simulink model "ILCadaptabledoble"  (R2023b)
settings: Solver=VariableStepAuto  StartTime=0.0  StopTime=25  RelTol=1e-3
values from neighbouring files (symbols this model uses):
  BL = 0.00223579    [ILCadaptable.m]    (also in parametros3.m)
  C1 = [1 0 0 0]    [ILCadaptable.m]    (also in parametros3.m = [1 0 0 0 0 0])
  C2 = [0 1 0 0]    [ILCadaptable.m]    (also in parametros3.m = [0 0 1 0 0 0])
  C3 = [0 0 1 0]    [ILCadaptable.m]    (also in parametros3.m = [0 0 0 0 1 0])
  C4 = [0 0 0 1]    [ILCadaptable.m]
  ek1_1 = out.ek1    [ILCadaptable.m]    (also in parametros3.m)
  ek2_1 = out.ek2    [ILCadaptable.m]    (also in parametros3.m)
  JL = 0.00040095    [ILCadaptable.m]    (also in parametros3.m)
  KB = 0.23351629    [ILCadaptable.m]    (also in parametros3.m)
  KD = 5    [ILCadaptable.m]
  KM = 0.23351629    [ILCadaptable.m]    (also in parametros3.m)
  L1 = 2    [ILCadaptable.m]    (also in parametros3.m)
  L2 = 2    [ILCadaptable.m]    (also in parametros3.m)
  LC = 0.0015    [ILCadaptable.m]    (also in parametros3.m)
  RC = 3.4    [ILCadaptable.m]    (also in parametros3.m)
  rt = 10    [ILCadaptable.m]    (also in parametros3.m)
libraries: simulink x2, slpidlib x2
settings Model: Creator=LENOVO  LastModifiedBy=LENOVO

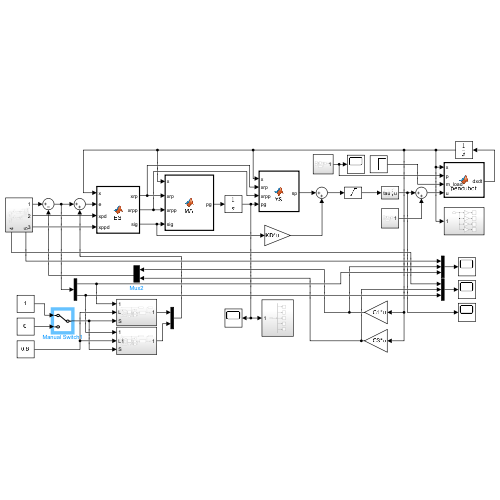
[thumbnail: Simulink's stored preview of the top-level diagram]
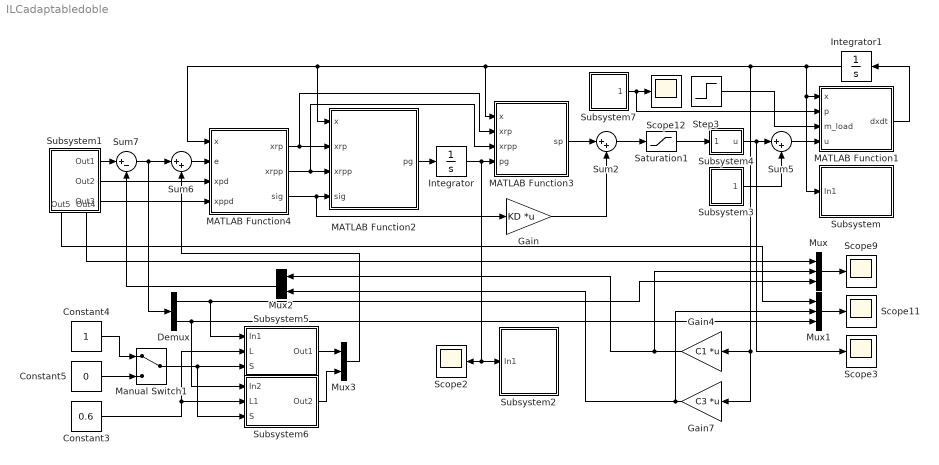
== system ILCadaptabledoble ==
  Constant3 : Constant  Value=0.6
  Constant4 : Constant
  Constant5 : Constant  Value=0
  Demux : Demux  Outputs=2
  Gain : Gain  Gain=KD  Multiplication=Matrix(K*u)
  Gain4 : Gain  Gain=C1  Multiplication=Matrix(K*u)
  Gain7 : Gain  Gain=C3  Multiplication=Matrix(K*u)
  Integrator : Integrator  InitialCondition=[0 0 0 0 0]
  Integrator1 : Integrator  InitialCondition=[-pi/2;0;0;0]
  MATLAB Function1 : MATLAB Function  TreatAsAtomicUnit=on
  MATLAB Function2 : MATLAB Function  TreatAsAtomicUnit=on
  MATLAB Function3 : MATLAB Function  TreatAsAtomicUnit=on
  MATLAB Function4 : MATLAB Function  TreatAsAtomicUnit=on
  Manual Switch1 : ManualSwitch
  Mux : Mux  Inputs=3
  Mux1 : Mux  Inputs=3
  Mux2 : Mux  Inputs=2
  Mux3 : Mux  Inputs=2
  Saturation1 : Saturate  UpperLimit=10  LowerLimit=-10
  Scope{2..3,9,11..12} (5 alike) : Scope
  Step3 : Step  Time=10  After=2  SampleTime=0
  Subsystem : Subsystem
  Subsystem1 : Subsystem
      settings: PortSchema="{\"entries\":[{\"content\":{\"sides\":[{\"content\":{},\"type\":\"ConnectorPlacement.EquallySpacedRectSide\",\"uuid\":\"9b7d0a68-027c-45ca-820c-f278bc6f32a7\"},{\"content\":{\"connectorIds\":[\"Out1\",\"Out2\",\"Out3\"],\"side\":\"RIGHT\"},\"type\":\"ConnectorPlacement.EquallySpacedRectSide\",\"uuid\":\"fa53ec67-4df6-4868-87ee-3d32a2fc1068\"},{\"content\":{\"side\":\"TOP\"},\"type\":\"ConnectorPlacement.EquallySpacedRectSide\",\"uuid\":\"8fcd41cb-9cc9-4cf7-b08f-50ea27c8effa\"},{\"content\":{\"connectorIds\":[\"Out4\",\"Out5\"],\"side\":\"BOTTOM\"},\"type\":\"ConnectorPlacement.EquallySpacedRectSide\",\"uuid\":\"53ef6b28-bc02-4c26-b41f-4cbf5a6224bd\"}]},\"type\":\"ConnectorPlacement.EquallySpacedConnector\",\"uuid\":\"01489902-74b8-4eba-a27b-b5ca226e6d88\"}],\"packageUris\":[\"http://schema.mathworks.com/mf0/Connector/R2020b\"],\"version\":\"1.0\"}"
  Subsystem2 : Subsystem
  Subsystem3 : Subsystem
  Subsystem4 : Subsystem
  Subsystem5 : Subsystem
  Subsystem6 : Subsystem
  Subsystem7 : Subsystem
  Sum2 : Sum  Inputs=|++
  Sum5 : Sum  Inputs=|++
  Sum6 : Sum  Inputs=|++
  Sum7 : Sum  Inputs=|+-
  wires:
  Saturation1/1 -> Subsystem4/1(tau)
  Step3/1 -> MATLAB Function1/3(m_load)
  Gain/1 -> Sum2/2
  MATLAB Function4/3(sig) -> Gain/1, MATLAB Function2/4(sig)
  Sum5/1 -> MATLAB Function1/4(u)
  Sum2/1 -> Saturation1/1
  Subsystem1/5(Out4) -> Mux/1
  Subsystem4/1(u) -> Scope3/1, Sum5/1
  MATLAB Function4/1(xrp) -> MATLAB Function2/2(xrp), MATLAB Function3/2(xrp)
  Mux/1 -> Scope9/1
  Mux1/1 -> Scope11/1
  Subsystem1/2(Out2) -> MATLAB Function4/3(xpd)
  MATLAB Function4/2(xrpp) -> MATLAB Function3/3(xrpp), MATLAB Function2/3(xrpp)
  MATLAB Function1/1(dxdt) -> Integrator1/1
  MATLAB Function3/1(sp) -> Sum2/1
  MATLAB Function2/1(pg) -> Integrator/1
  Subsystem1/4(Out5) -> Mux1/1
  Subsystem1/3(Out3) -> MATLAB Function4/4(xppd)
  Integrator1/1 -> Subsystem/1(In1), MATLAB Function1/1(x), Gain7/1, Gain4/1, MATLAB Function2/1(x), MATLAB Function4/1(x), MATLAB Function3/1(x)
  Integrator/1 -> Subsystem2/1(In1), Scope2/1, MATLAB Function3/4(pg)
  Sum6/1 -> MATLAB Function4/2(e)
  Sum7/1 -> Demux/1, Sum6/1
  Subsystem1/1(Out1) -> Sum7/1
  Constant4/1 -> Manual Switch1/1
  Constant5/1 -> Manual Switch1/2
  Constant3/1 -> Subsystem6/2(L1), Subsystem5/2(L)
  Manual Switch1/1 -> Subsystem6/3(S), Subsystem5/3(S)
  Demux/1 -> Subsystem5/1(In1), Mux/3
  Demux/2 -> Subsystem6/1(In2), Mux1/3
  Mux2/1 -> Sum7/2
  Subsystem5/1(Out1) -> Mux3/1
  Subsystem6/1(Out2) -> Mux3/2
  Mux3/1 -> Sum6/2
  Subsystem7/1(Out1) -> MATLAB Function1/2(p), Scope12/1
  Gain4/1 -> Mux/2, Mux2/1
  Gain7/1 -> Mux1/2, Mux2/2
  Subsystem3/1(Out2) -> Sum5/2

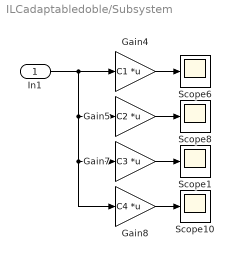
== system ILCadaptabledoble/Subsystem ==
  In1 : Inport
  Gain4 : Gain  Gain=C1  Multiplication=Matrix(K*u)
  Gain5 : Gain  Gain=C2  Multiplication=Matrix(K*u)
  Gain7 : Gain  Gain=C3  Multiplication=Matrix(K*u)
  Gain8 : Gain  Gain=C4  Multiplication=Matrix(K*u)
  Scope{1,6,8,10} (4 alike) : Scope
  wires:
  In1/1 -> Gain8/1, Gain7/1, Gain5/1, Gain4/1
  Gain4/1 -> Scope6/1
  Gain5/1 -> Scope8/1
  Gain7/1 -> Scope1/1
  Gain8/1 -> Scope10/1

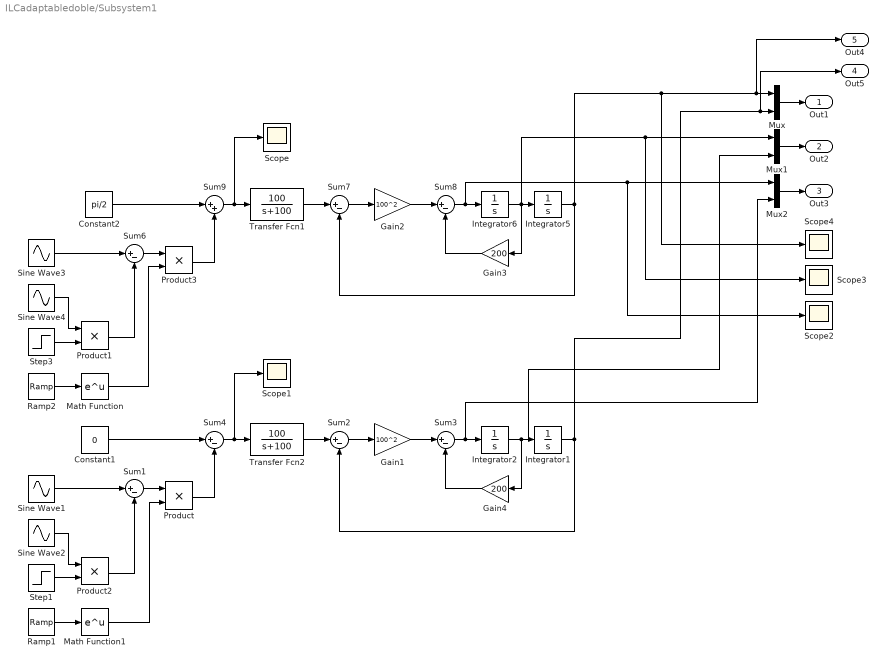
== system ILCadaptabledoble/Subsystem1 ==
  Constant1 : Constant  Value=0
  Constant2 : Constant  Value=pi/2
  Gain1 : Gain  Gain=100^2
  Gain2 : Gain  Gain=100^2
  Gain3 : Gain  Gain=200
  Gain4 : Gain  Gain=200
  Integrator{1..2,5..6} (4 alike) : Integrator
  Math Function : Math
  Math Function1 : Math
  Mux : Mux  Inputs=2
  Mux1 : Mux  Inputs=2
  Mux2 : Mux  Inputs=2
  Product{,1..3} (4 alike) : Product
  Ramp1 : simulink/Sources/Ramp  slope=0  start=10  InitialOutput=0
  Ramp2 : simulink/Sources/Ramp  slope=0  start=10  InitialOutput=0
  Scope{,1..4} (5 alike) : Scope
  Sine Wave1 : Sin  Amplitude=1.4  Frequency=2  SampleTime=0
  Sine Wave2 : Sin  Amplitude=1.4  Frequency=5  SampleTime=0
  Sine Wave3 : Sin  Amplitude=1.4  Frequency=2  SampleTime=0
  Sine Wave4 : Sin  Amplitude=1.4  Frequency=5  SampleTime=0
  Step1 : Step  Time=0  After=0  SampleTime=0
  Step3 : Step  Time=0  After=0  SampleTime=0
  Sum{1..4,6..8} (7 alike) : Sum  Inputs=|+-
  Sum9 : Sum  Inputs=|++
  Transfer Fcn1 : TransferFcn  Numerator=[100]  Denominator=[1 100]
  Transfer Fcn2 : TransferFcn  Numerator=[100]  Denominator=[1 100]
  Out1 : Outport
  Out2 : Outport  Port=2
  Out3 : Outport  Port=3
  Out5 : Outport  Port=4
  Out4 : Outport  Port=5
  wires:
  Mux/1 -> Out1/1
  Mux1/1 -> Out2/1
  Mux2/1 -> Out3/1
  Integrator5/1 -> Scope4/1, Out4/1, Mux/1, Sum7/2
  Sine Wave3/1 -> Sum6/1
  Sum7/1 -> Gain2/1
  Sum8/1 -> Scope2/1, Mux2/1, Integrator6/1
  Sine Wave4/1 -> Product1/1
  Gain2/1 -> Sum8/1
  Transfer Fcn1/1 -> Sum7/1
  Gain3/1 -> Sum8/2
  Product1/1 -> Sum6/2
  Step3/1 -> Product1/2
  Constant2/1 -> Sum9/1
  Integrator6/1 -> Scope3/1, Mux1/1, Gain3/1, Integrator5/1
  Sum9/1 -> Scope/1, Transfer Fcn1/1
  Sum4/1 -> Scope1/1, Transfer Fcn2/1
  Sum3/1 -> Mux2/2, Integrator2/1
  Gain1/1 -> Sum3/1
  Transfer Fcn2/1 -> Sum2/1
  Sum2/1 -> Gain1/1
  Step1/1 -> Product2/2
  Constant1/1 -> Sum4/1
  Integrator1/1 -> Out5/1, Mux/2, Sum2/2
  Sine Wave1/1 -> Sum1/1
  Gain4/1 -> Sum3/2
  Integrator2/1 -> Mux1/2, Gain4/1, Integrator1/1
  Product2/1 -> Sum1/2
  Sine Wave2/1 -> Product2/1
  Math Function/1 -> Product3/2
  Math Function1/1 -> Product/2
  Ramp2/1 -> Math Function/1
  Ramp1/1 -> Math Function1/1
  Sum6/1 -> Product3/1
  Product3/1 -> Sum9/2
  Sum1/1 -> Product/1
  Product/1 -> Sum4/2

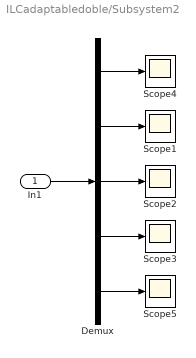
== system ILCadaptabledoble/Subsystem2 ==
  In1 : Inport
  Demux : Demux  Outputs=5
  Scope{1..5} (5 alike) : Scope
  wires:
  In1/1 -> Demux/1
  Demux/3 -> Scope2/1
  Demux/2 -> Scope1/1
  Demux/1 -> Scope4/1
  Demux/4 -> Scope3/1
  Demux/5 -> Scope5/1

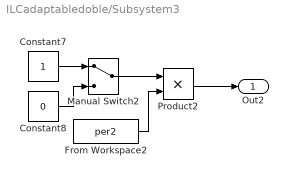
== system ILCadaptabledoble/Subsystem3 ==
  Constant7 : Constant
  Constant8 : Constant  Value=0
  From Workspace2 : FromWorkspace  VariableName=per2
  Manual Switch2 : ManualSwitch
  Product2 : Product
  Out2 : Outport
  wires:
  Product2/1 -> Out2/1
  From Workspace2/1 -> Product2/2
  Constant7/1 -> Manual Switch2/1
  Constant8/1 -> Manual Switch2/2
  Manual Switch2/1 -> Product2/1

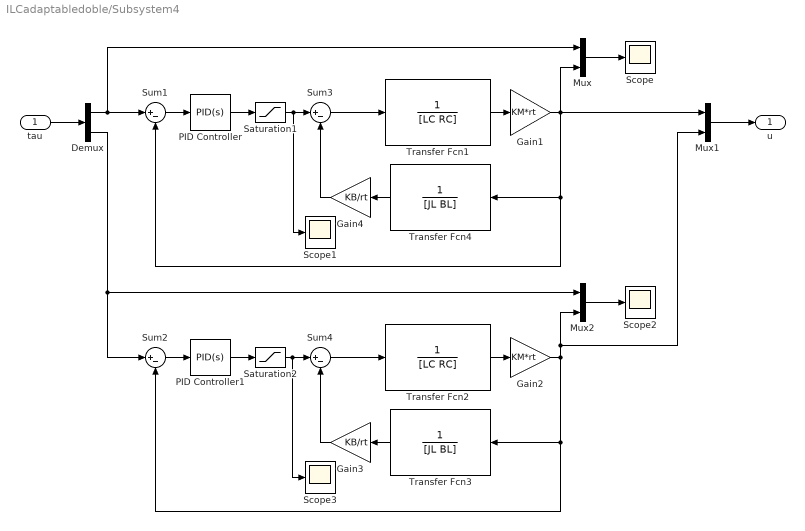
== system ILCadaptabledoble/Subsystem4 ==
  tau : Inport
  Demux : Demux  Outputs=2
  Gain1 : Gain  Gain=KM*rt
  Gain2 : Gain  Gain=KM*rt
  Gain3 : Gain  Gain=KB/rt
  Gain4 : Gain  Gain=KB/rt
  Mux : Mux  Inputs=2
  Mux1 : Mux  Inputs=2
  Mux2 : Mux  Inputs=2
  PID Controller : slpidlib/PID Controller  Controller=PID  Form=Parallel  TimeDomain=Continuous-time  UseExternalTs=off  SampleTime=-1  IntegratorMethod=Forward Euler  FilterMethod=Forward Euler  ControllerParametersSource=internal  P=100  I=50  UseKiTs=off  D=20  N=100  UseFilter=on  TunerSelectOption=Transfer Function Based (PID Tuner App)  InitialConditionSource=internal  InitialConditionForIntegrator=0  InitialConditionForFilter=0  DifferentiatorICPrevScaledInput=0  ExternalReset=none  TrackingMode=off  Kt=1  LimitOutput=off  SatLimitsSource=internal  UpperSaturationLimit=inf  LowerSaturationLimit=-inf  LinearizeAsGain=on  AntiWindupMode=none  Kb=1  LimitIntegrator=off  UpperIntegratorSaturationLimit=inf  LowerIntegratorSaturationLimit=-inf  POutMin=[]  POutMax=[]  IOutMin=[]  IOutMax=[]  DOutMin=[]  DOutMax=[]  NOutMin=[]  NOutMax=[]  SumOutMin=[]  SumOutMax=[]  SaturationOutMin=[]  SaturationOutMax=[]  PParamMin=[]  PParamMax=[]  IParamMin=[]  IParamMax=[]  DParamMin=[]  DParamMax=[]  NParamMin=[]  NParamMax=[]  KbParamMin=[]  KbParamMax=[]  KtParamMin=[]  KtParamMax=[]  KbOutMin=[]  KbOutMax=[]  KtOutMin=[]  KtOutMax=[]  IntegratorOutMin=[]  IntegratorOutMax=[]  FilterOutMin=[]  FilterOutMax=[]  SumI1OutMin=[]  SumI1OutMax=[]  SumI2OutMin=[]  SumI2OutMax=[]  SumI3OutMin=[]  SumI3OutMax=[]  SumI4OutMin=[]  SumI4OutMax=[]  SumDOutMin=[]  SumDOutMax=[]  DifferentiatorOutMin=[]  DifferentiatorOutMax=[]  FilterDiffOutCoefMin=[]  FilterDiffOutCoefMax=[]  ReciprocalOutMin=[]  ReciprocalOutMax=[]  SumDenOutMin=[]  SumDenOutMax=[]  SumNumOutMin=[]  SumNumOutMax=[]  DivideOutMin=[]  DivideOutMax=[]  UdiffTsProdOutMin=[]  UdiffTsProdOutMax=[]  NTsProdOutMin=[]  NTsProdOutMax=[]  UintegralTsProdOutMin=[]  UintegralTsProdOutMax=[]  UngainTsProdOutMin=[]  UngainTsProdOutMax=[]  ClampingZeroOutDataTypeStr=Inherit: Inherit via back propagation  ClampingZeroOutMin=[]  ClampingZeroOutMax=[]  FilterDenConstantOutDataTypeStr=Inherit: Inherit via back propagation  FilterDenConstantOutMin=[]  FilterDenConstantOutMax=[]  PCopyOutDataTypeStr=Inherit: Inherit via back propagation  PCopyOutMin=[]  PCopyOutMax=[]  NCopyOutDataTypeStr=Inherit: Inherit via back propagation  NCopyOutMin=[]  NCopyOutMax=[]  IntegratorContinuousStateAttributes=''  IntegratorStateMustResolveToSignalObject=off  IntegratorRTWStateStorageClass=Auto  FilterContinuousStateAttributes=''  FilterStateMustResolveToSignalObject=off  FilterRTWStateStorageClass=Auto  ParallelPVariant=InternalParameters  IdealPVariant=Disabled  IVariant=InternalParameters  DVariant=InternalParameters  IntegratorVariant=Continuous  SatVariant=Disabled  AWVariant=Passthrough  PCopyVariant=Disabled  TRVariant=Disabled  FdbkBlocksVariant=Forward  IdealPFdbkVariant=Disabled  SatFdbkVariant=Disabled  DerivativeFilterVariant=ContFilter  NVariant=InternalParameters  NCopyVariant=Disabled  FilterICVariant=InternalICsFilter  IntegratorICVariant=InternalICs  ExternalResetVariant=Disabled  TRSumVariant=Passthrough  SumFdbkVariant=Disabled  SumVariant=Sum_PID  TsampFilterVariant=InternalTs  TsampNgainVariant=Passthrough  TsampIntegralVariant=Disabled_SignalSpec  ExternalSaturationOutDataTypeStr=Inherit: Same as second input
  PID Controller1 : slpidlib/PID Controller  Controller=PID  Form=Parallel  TimeDomain=Continuous-time  UseExternalTs=off  SampleTime=-1  IntegratorMethod=Forward Euler  FilterMethod=Forward Euler  ControllerParametersSource=internal  P=100  I=50  UseKiTs=off  D=20  N=100  UseFilter=on  TunerSelectOption=Transfer Function Based (PID Tuner App)  InitialConditionSource=internal  InitialConditionForIntegrator=0  InitialConditionForFilter=0  DifferentiatorICPrevScaledInput=0  ExternalReset=none  TrackingMode=off  Kt=1  LimitOutput=off  SatLimitsSource=internal  UpperSaturationLimit=inf  LowerSaturationLimit=-inf  LinearizeAsGain=on  AntiWindupMode=none  Kb=1  LimitIntegrator=off  UpperIntegratorSaturationLimit=inf  LowerIntegratorSaturationLimit=-inf  POutMin=[]  POutMax=[]  IOutMin=[]  IOutMax=[]  DOutMin=[]  DOutMax=[]  NOutMin=[]  NOutMax=[]  SumOutMin=[]  SumOutMax=[]  SaturationOutMin=[]  SaturationOutMax=[]  PParamMin=[]  PParamMax=[]  IParamMin=[]  IParamMax=[]  DParamMin=[]  DParamMax=[]  NParamMin=[]  NParamMax=[]  KbParamMin=[]  KbParamMax=[]  KtParamMin=[]  KtParamMax=[]  KbOutMin=[]  KbOutMax=[]  KtOutMin=[]  KtOutMax=[]  IntegratorOutMin=[]  IntegratorOutMax=[]  FilterOutMin=[]  FilterOutMax=[]  SumI1OutMin=[]  SumI1OutMax=[]  SumI2OutMin=[]  SumI2OutMax=[]  SumI3OutMin=[]  SumI3OutMax=[]  SumI4OutMin=[]  SumI4OutMax=[]  SumDOutMin=[]  SumDOutMax=[]  DifferentiatorOutMin=[]  DifferentiatorOutMax=[]  FilterDiffOutCoefMin=[]  FilterDiffOutCoefMax=[]  ReciprocalOutMin=[]  ReciprocalOutMax=[]  SumDenOutMin=[]  SumDenOutMax=[]  SumNumOutMin=[]  SumNumOutMax=[]  DivideOutMin=[]  DivideOutMax=[]  UdiffTsProdOutMin=[]  UdiffTsProdOutMax=[]  NTsProdOutMin=[]  NTsProdOutMax=[]  UintegralTsProdOutMin=[]  UintegralTsProdOutMax=[]  UngainTsProdOutMin=[]  UngainTsProdOutMax=[]  ClampingZeroOutDataTypeStr=Inherit: Inherit via back propagation  ClampingZeroOutMin=[]  ClampingZeroOutMax=[]  FilterDenConstantOutDataTypeStr=Inherit: Inherit via back propagation  FilterDenConstantOutMin=[]  FilterDenConstantOutMax=[]  PCopyOutDataTypeStr=Inherit: Inherit via back propagation  PCopyOutMin=[]  PCopyOutMax=[]  NCopyOutDataTypeStr=Inherit: Inherit via back propagation  NCopyOutMin=[]  NCopyOutMax=[]  IntegratorContinuousStateAttributes=''  IntegratorStateMustResolveToSignalObject=off  IntegratorRTWStateStorageClass=Auto  FilterContinuousStateAttributes=''  FilterStateMustResolveToSignalObject=off  FilterRTWStateStorageClass=Auto  ParallelPVariant=InternalParameters  IdealPVariant=Disabled  IVariant=InternalParameters  DVariant=InternalParameters  IntegratorVariant=Continuous  SatVariant=Disabled  AWVariant=Passthrough  PCopyVariant=Disabled  TRVariant=Disabled  FdbkBlocksVariant=Forward  IdealPFdbkVariant=Disabled  SatFdbkVariant=Disabled  DerivativeFilterVariant=ContFilter  NVariant=InternalParameters  NCopyVariant=Disabled  FilterICVariant=InternalICsFilter  IntegratorICVariant=InternalICs  ExternalResetVariant=Disabled  TRSumVariant=Passthrough  SumFdbkVariant=Disabled  SumVariant=Sum_PID  TsampFilterVariant=InternalTs  TsampNgainVariant=Passthrough  TsampIntegralVariant=Disabled_SignalSpec  ExternalSaturationOutDataTypeStr=Inherit: Same as second input
  Saturation1 : Saturate  UpperLimit=250  LowerLimit=-250
  Saturation2 : Saturate  UpperLimit=250  LowerLimit=-250
  Scope{,1..3} (4 alike) : Scope
  Sum{1..4} (4 alike) : Sum  Inputs=|+-
  Transfer Fcn1 : TransferFcn  Denominator=[LC RC]
  Transfer Fcn2 : TransferFcn  Denominator=[LC RC]
  Transfer Fcn3 : TransferFcn  Denominator=[JL BL]
  Transfer Fcn4 : TransferFcn  Denominator=[JL BL]
  u : Outport
  wires:
  tau/1 -> Demux/1
  Demux/1 -> Sum1/1, Mux/1
  Mux/1 -> Scope/1
  Sum1/1 -> PID Controller/1
  Transfer Fcn1/1 -> Gain1/1
  Gain1/1 -> Sum1/2, Transfer Fcn4/1, Mux1/1, Mux/2
  Gain4/1 -> Sum3/2
  Sum3/1 -> Transfer Fcn1/1
  Transfer Fcn4/1 -> Gain4/1
  Mux1/1 -> u/1
  PID Controller/1 -> Saturation1/1
  PID Controller1/1 -> Saturation2/1
  Sum2/1 -> PID Controller1/1
  Demux/2 -> Sum2/1, Mux2/1
  Transfer Fcn2/1 -> Gain2/1
  Transfer Fcn3/1 -> Gain3/1
  Gain3/1 -> Sum4/2
  Gain2/1 -> Mux2/2, Mux1/2, Sum2/2, Transfer Fcn3/1
  Mux2/1 -> Scope2/1
  Sum4/1 -> Transfer Fcn2/1
  Saturation1/1 -> Scope1/1, Sum3/1
  Saturation2/1 -> Scope3/1, Sum4/1

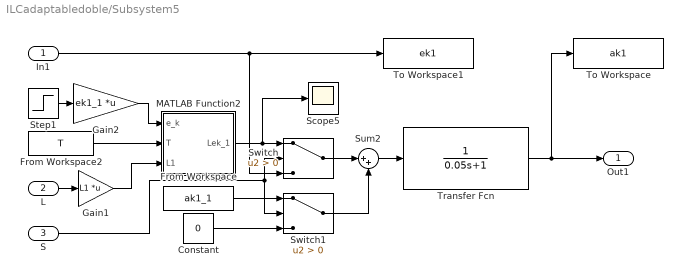
== system ILCadaptabledoble/Subsystem5 ==
  In1 : Inport
  L : Inport  Port=2
  S : Inport  Port=3
  Constant : Constant  Value=0
  From Workspace : FromWorkspace  VariableName=ak1_1
  From Workspace2 : FromWorkspace  VariableName=T
  Gain1 : Gain  Gain=L1  Multiplication=Matrix(K*u)
  Gain2 : Gain  Gain=ek1_1  Multiplication=Matrix(K*u)
  MATLAB Function2 : MATLAB Function  TreatAsAtomicUnit=on
  Scope5 : Scope
  Step1 : Step  Time=0  SampleTime=0
  Sum2 : Sum  Inputs=|++
  Switch : Switch  Criteria=u2 > Threshold  SaturateOnIntegerOverflow=off  InputSameDT=off
  Switch1 : Switch  Criteria=u2 > Threshold  SaturateOnIntegerOverflow=off  InputSameDT=off
  To Workspace : ToWorkspace  VariableName=ak1  SampleTime=-1
  To Workspace1 : ToWorkspace  VariableName=ek1  SampleTime=-1
  Transfer Fcn : TransferFcn  Denominator=[0.05 1]
  Out1 : Outport
  wires:
  From Workspace2/1 -> MATLAB Function2/2(T)
  In1/1 -> Switch/3, To Workspace1/1
  Gain2/1 -> MATLAB Function2/1(e_k)
  Step1/1 -> Gain2/1
  Constant/1 -> Switch1/3
  MATLAB Function2/1(Lek_1) -> Scope5/1, Switch/1
  Sum2/1 -> Transfer Fcn/1
  Switch1/1 -> Sum2/2
  From Workspace/1 -> Switch1/1
  Switch/1 -> Sum2/1
  Transfer Fcn/1 -> To Workspace/1, Out1/1
  L/1 -> Gain1/1
  S/1 -> Switch1/2, Switch/2
  Gain1/1 -> MATLAB Function2/3(L1)

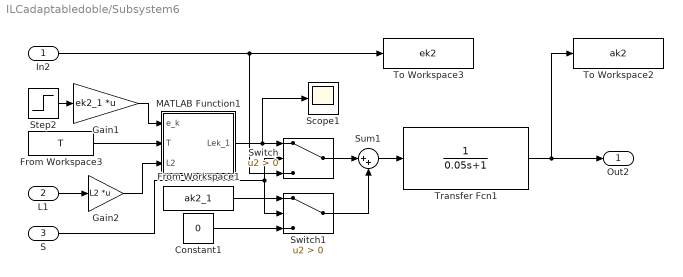
== system ILCadaptabledoble/Subsystem6 ==
  In2 : Inport
  L1 : Inport  Port=2
  S : Inport  Port=3
  Constant1 : Constant  Value=0
  From Workspace1 : FromWorkspace  VariableName=ak2_1
  From Workspace3 : FromWorkspace  VariableName=T
  Gain1 : Gain  Gain=ek2_1  Multiplication=Matrix(K*u)
  Gain2 : Gain  Gain=L2  Multiplication=Matrix(K*u)
  MATLAB Function1 : MATLAB Function  TreatAsAtomicUnit=on
  Scope1 : Scope
  Step2 : Step  Time=0  SampleTime=0
  Sum1 : Sum  Inputs=|++
  Switch : Switch  Criteria=u2 > Threshold  SaturateOnIntegerOverflow=off  InputSameDT=off
  Switch1 : Switch  Criteria=u2 > Threshold  SaturateOnIntegerOverflow=off  InputSameDT=off
  To Workspace2 : ToWorkspace  VariableName=ak2  SampleTime=-1
  To Workspace3 : ToWorkspace  VariableName=ek2  SampleTime=-1
  Transfer Fcn1 : TransferFcn  Denominator=[0.05 1]
  Out2 : Outport
  wires:
  MATLAB Function1/1(Lek_1) -> Scope1/1, Switch/1
  S/1 -> Switch1/2, Switch/2
  Sum1/1 -> Transfer Fcn1/1
  Gain1/1 -> MATLAB Function1/1(e_k)
  Transfer Fcn1/1 -> To Workspace2/1, Out2/1
  In2/1 -> Switch/3, To Workspace3/1
  From Workspace1/1 -> Switch1/1
  From Workspace3/1 -> MATLAB Function1/2(T)
  Constant1/1 -> Switch1/3
  Step2/1 -> Gain1/1
  Switch1/1 -> Sum1/2
  Switch/1 -> Sum1/1
  L1/1 -> Gain2/1
  Gain2/1 -> MATLAB Function1/3(L2)

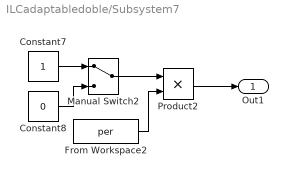
== system ILCadaptabledoble/Subsystem7 ==
  Constant7 : Constant
  Constant8 : Constant  Value=0
  From Workspace2 : FromWorkspace  VariableName=per
  Manual Switch2 : ManualSwitch
  Product2 : Product
  Out1 : Outport
  wires:
  Product2/1 -> Out1/1
  Constant8/1 -> Manual Switch2/2
  Constant7/1 -> Manual Switch2/1
  Manual Switch2/1 -> Product2/1
  From Workspace2/1 -> Product2/2

== matlab function ILCadaptabledoble/MATLAB Function1 ==
  data: x input; p input; m_load input; u input; dxdt output
function dxdt = pendubot(x,p,m_load,u)

%definición de parametros
m1 = 0.066+p(1)+m_load;
m2 = 0.0792+p(2);
l1 = 0.25+p(3);
l2 = 0.3+p(4);
lc1 = l1/2;
lc2 = l2/2;
I1 = 0.00138+p(5);
I2 = 0.00238+p(6);
g = 9.81;

%calculo de las constantes del sistema
a1 = m1*lc1^2+m2*l1^2+I1;
a2 = m2*lc2^2+I2;
a3 = m2*l1*lc2;
a4 = m1*lc1+m2*l1;
a5 = m2*lc2;

%variables de estado
x1 = x(1);
x2 = x(2);
x3 = x(3);
x4 = x(4);

%Matrices del sistema
G = [a4*g*cos(x1)+a5*g*cos(x1+x3);a5*g*cos(x1+x3)];%matriz de gravedad 
C = [-2*a3*sin(x3)*x4 -a3*sin(x3)*x4;
     a3*sin(x3)*x2 0];%matriz de velocidad o coriolis
M = [a1+a2+2*a3*cos(x3) a2+a3*cos(x3);
     a2+a3*cos(x3) a2];%matriz de aceleración

%d/dt[x1;x2;x3;x4]=[f1;f2;f3;f4]
%calculo de f2 y f4 
xb = M^(-1)*u-M^(-1)*C*[x2;x4]-M^(-1)*G;

%sistema en la forma d/dt[x1;x2;x3;x4]=[f1;f2;f3;f4] 
dxdt = [x2; 
        xb(1);
        x4;
        xb(2)];

== matlab function ILCadaptabledoble/MATLAB Function3 ==
  data: x input; xrp input; xrpp input; pg input; sp output
function sp = YS(x,xrp,xrpp,pg)

%variables de estado
x1 = x(1);
x2 = x(2);
x3 = x(3);
x4 = x(4);

%Matriz Y(x,xr) equivalente
Y = [xrpp(1),xrpp(1)+xrpp(2),cos(x3)*xrpp(1)+cos(x3)*xrpp(2)-2*sin(x3)*x4*xrp(1)-sin(x3)*x4*xrp(2),cos(x3),cos(x1+x3);0,xrpp(1)+xrpp(2),cos(x3)*xrpp(1)+sin(x3)*x2*xrp(1),0,cos(x1+x3)];

%acción de control final
sp = Y*pg

== matlab function ILCadaptabledoble/MATLAB Function2 ==
  data: x input; xrp input; xrpp input; sig input; pg output
function pg = MA(x,xrp,xrpp,sig)

%variables de estado
x1 = x(1);
x2 = x(2);
x3 = x(3);
x4 = x(4);

%Matriz Y(x,xr) equivalente
Y = [xrpp(1),xrpp(1)+xrpp(2),cos(x3)*xrpp(1)+cos(x3)*xrpp(2)-2*sin(x3)*x4*xrp(1)-sin(x3)*x4*xrp(2),cos(x3),cos(x1+x3);0,xrpp(1)+xrpp(2),cos(x3)*xrpp(1)+sin(x3)*x2*xrp(1),0,cos(x1+x3)];

%Ganancia Kpi de parametros
Kpi = 10000*[1 0 0 0 0;0 1 0 0 0;0 0 1 0 0;0 0 0 1 0;0 0 0 0 1]

%acción de control
pg = Kpi^(-1)*Y'*sig

== matlab function ILCadaptabledoble/MATLAB Function4 ==
  data: x input; e input; xpd input; xppd input; xrp output; xrpp output; sig output
function [xrp,xrpp,sig] = ES(x,e,xpd,xppd)

%variables de estado
xv = [x(2);x(4)];

%Ganancia del error de segumiento
A = 2*[1 0;0 1];

%Calculo de velocidad y aceleración de referencia
xgp = xpd-xv;

xrp = xpd+A*e;
xrpp = xppd+A*xgp;

%error de seguimiento
sig = xrp-xv

== matlab function ILCadaptabledoble/Subsystem5/MATLAB Function2 ==
  data: Lek_1 output; e_k input; T input; L1 input
function Lek_1 = noncausal(e_k,T,L1)
n = int32(T);
dt = 0.05;
d1x = (e_k(n+1)-e_k(n))/dt;
d2x = (e_k(n+2)-2*e_k(n+1)+e_k(n))/dt;
d3x = (e_k(n+3)-3*e_k(n+2)+3*e_k(n+1)-e_k(n))/dt;
d4x = (e_k(n+4)-4*e_k(n+3)+6*e_k(n+2)-4*e_k(n+1)+e_k(n))/dt;
d5x = (e_k(n+5)-5*e_k(n+4)+10*e_k(n+3)-10*e_k(n+2)+5*e_k(n+1)-e_k(n))/dt;

Lek_1 = L1*(0.01*d5x+0.02*d4x+0.05*d3x+0.1*d2x+0.5*d1x+e_k(n));

== matlab function ILCadaptabledoble/Subsystem6/MATLAB Function1 ==
  data: Lek_1 output; e_k input; T input; L2 input
function Lek_1 = noncausal(e_k,T,L2)
n = int32(T);
dt = 0.05;
d1x = (e_k(n+1)-e_k(n))/dt;
d2x = (e_k(n+2)-2*e_k(n+1)+e_k(n))/dt;
d3x = (e_k(n+3)-3*e_k(n+2)+3*e_k(n+1)-e_k(n))/dt;
d4x = (e_k(n+4)-4*e_k(n+3)+6*e_k(n+2)-4*e_k(n+1)+e_k(n))/dt;
d5x = (e_k(n+5)-5*e_k(n+4)+10*e_k(n+3)-10*e_k(n+2)+5*e_k(n+1)-e_k(n))/dt;

Lek_1 = L2*(0.01*d5x+0.02*d4x+0.05*d3x+0.1*d2x+0.5*d1x+e_k(n));
